simulink model "ControleLateralApplication_atual"  (R2023b)
settings: Solver=ode23tb  StartTime=0.0  StopTime=TME.Simulation  FixedStep=.001  RelTol=2e-1  EnableMultiTasking=on
StartFcn:
  | %tic
StopFcn:
  | %toc
model workspace (MAT data in the model file):
  A_mu = 10
  B_reff = 8.386
  Cz = 7766.25
  DCT_Param : object (value not decoded)
  DLCXref = [0 6 7 14 33.5 34 42 50 60]
  DLCYref = [0 0 -4.5 -4 -3.75 1.5 0.5 0 0]
  D_reff = 0.25826
  Downshift_Speeds = [9.5625 12.9375 16.3125 19.6875 23.0625 26.4375 29.8125 33.1875 36.5625 39.9375 43.3125 46.6875 ... (28 elements, 4x7)]
  EngRevLim = 7000
  Pedal_Positions = [0.1 0.4 0.5 0.9]
  SUS : object (value not decoded)
  Upshift_Speeds = [12.9375 16.3125 19.6875 33 26.4375 29.8125 33.1875 52.5 39.9375 43.3125 46.6875 77.25 ... (28 elements, 4x7)]
  VEH : object (value not decoded)
  V_o = 16.7
  V_xlow = 1
  WH : object (value not decoded)
  a = 1.4
  alpha_max = 1.5
  alpha_min = -1.5
  b = 1.8
  c_zo = 209651
  epsilon = 0.1
  h = 0.134
  path : object (value not decoded)
  pio = 220000
  q_Fcx = 0
  q_Fz2 = 15.4
  q_Fzy = 0
  q_reo = 0.9974
  q_sx1 = -0.007764
  q_sx10 = 0.2824
  q_sx11 = 5.349
  q_sx12 = 0
  q_sx13 = 0
  q_sx14 = 0
  q_sx2 = 1.1915
  q_sx3 = 0.013948
  q_sx4 = 4.912
  q_sx5 = 1.02
  q_sx6 = 22.83
  q_sx7 = 0.7104
  q_sx8 = -0.023393
  q_sx9 = 0.6581
  q_sy1 = 0.00702
  q_sy2 = 0
  q_sy3 = 0.001515
  q_sy4 = 8.514e-05
  q_sy5 = 0
  q_sy6 = 0
  q_sy7 = 0.9008
  q_sy8 = -0.4089
  q_v1 = 0.0007742
  q_v2 = 0.04667
  r_Bx1 = 12.531
  r_Bx2 = 9.532
  r_Bx3 = 0
  r_By1 = 10.615
  r_By2 = 7.705
  r_By3 = 3.433e-06
  r_By4 = 0
  r_Cx1 = 1.019
  r_Cy1 = 1.0585
  r_Ex1 = -0.4487
  r_Ex2 = -0.4726
  r_Ey1 = 0.3132
  r_Ey2 = 7.63e-06
  r_Hx1 = 0.0002374
  r_Hy1 = 0.011646
  r_Hy2 = 7.63e-06
  r_Vy1 = 0.05654
  r_Vy2 = 7.63e-06
  r_Vy3 = 0
  r_Vy4 = 99.9
  r_Vy5 = 2
  r_Vy6 = 15.814
  r_o = 0.3135
  vehWidth = 2
  w = 1
symbols that are objects in the model workspace (value not decoded): VEH
undefined symbols (not defined in the file): C1, C2, C3, Disabled, EV, GND, MTR, Right, SENSOR, STEER, WHL
libraries: autolibutils x5, vehdynlibscenariocommon x5, autolibshared x5, sim3dlib x4, vehdynlibtirecommon x2, autolibmappedmotor x2, vehdynlibviscommon x2, vehdynlibsteering x1, slpidlib x1, vehdynlibdriver x1, vehdynlibsens x1, sharedtransform x1
(part 6 of 6)

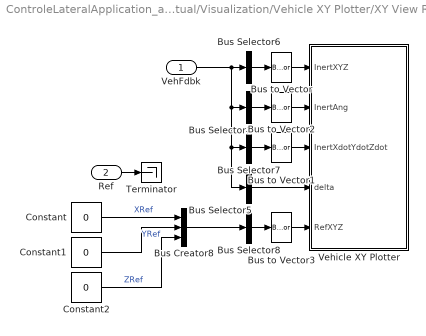
== system ControleLateralApplication_atual/Visualization/Vehicle XY Plotter/XY View Ref ==
  VehFdbk : Inport
  Ref : Inport  Port=2
  Bus Creator8 : BusCreator  Inputs=3
  Bus Selector1 : BusSelector  OutputSignals=Chassis.phi,Chassis.theta,Chassis.psi  OutputAsBus=on
  Bus Selector5 : BusSelector  OutputSignals=Driveline.WhlAng  OutputAsBus=on
  Bus Selector6 : BusSelector  OutputSignals=Chassis.GeomX,Chassis.GeomY,Chassis.GeomZ  OutputAsBus=on
  Bus Selector7 : BusSelector  OutputSignals=Chassis.GeomXdot,Chassis.GeomYdot,Chassis.GeomZdot  OutputAsBus=on
  Bus Selector8 : BusSelector  OutputSignals=XRef,YRef,ZRef  OutputAsBus=on
  Bus to Vector{,1..3} (4 alike) : BusToVector
  Constant : Constant  Value=0
  Constant1 : Constant  Value=0
  Constant2 : Constant  Value=0
  Terminator : Terminator
  Vehicle XY Plotter : Subsystem  mask(Vehicle XY Plotter){a=EV.FrontAxlePositionfromCG, b=EV.RearAxlePositionfromCG, w=EV.TrackWidth(1), figBorder=10, bufferSize=1024, extRef=on, pltDT=.1}
      mask prompts: a "Distance to front axle from CG, a [m]:"; b "Distance to rear axle from CG, b [m]:"; w "Track width, w [m]:"; figBorder "Distance to figure borders, figBorder [m]:"; bufferSize "Path buffer sampe size, bufferSize []:"; extRef "Plot path reference, extRef"; pltDT "Plot update rate, pltDT [s]:"
      mask help:
      | This block will display a MATLAB figure which indicates the vehicle path, current position and heading velocity.
      | An optional path reference is also provided.
      mask init: same as ControleLateralApplication_atual/Visualization/Vehicle XY Plotter/XY View/Vehicle XY Plotter
      mask TypeOptions a: Vehicle XY Plotter/a
      mask TypeOptions b: Vehicle XY Plotter/b
      mask TypeOptions w: Vehicle XY Plotter/w
      mask TypeOptions figBorder: Vehicle XY Plotter/figBorder
      mask TypeOptions bufferSize: Vehicle XY Plotter/bufferSize
  wires:
  Bus Selector8/1 -> Bus to Vector3/1
  Bus to Vector1/1 -> Vehicle XY Plotter/3(InertXdotYdotZdot)
  VehFdbk/1 -> Bus Selector5/1, Bus Selector7/1, Bus Selector1/1, Bus Selector6/1
  Bus Selector7/1 -> Bus to Vector1/1
  Bus Selector6/1 -> Bus to Vector/1
  Bus Selector1/1 -> Bus to Vector2/1
  Bus Selector5/1 -> Vehicle XY Plotter/4(delta)
  Bus to Vector/1 -> Vehicle XY Plotter/1(InertXYZ)
  Bus to Vector2/1 -> Vehicle XY Plotter/2(InertAng)
  Bus to Vector3/1 -> Vehicle XY Plotter/5(RefXYZ)
  Constant/1 -> Bus Creator8/1  "XRef"
  Constant1/1 -> Bus Creator8/2  "YRef"
  Constant2/1 -> Bus Creator8/3  "ZRef"
  Bus Creator8/1 -> Bus Selector8/1
  Ref/1 -> Terminator/1

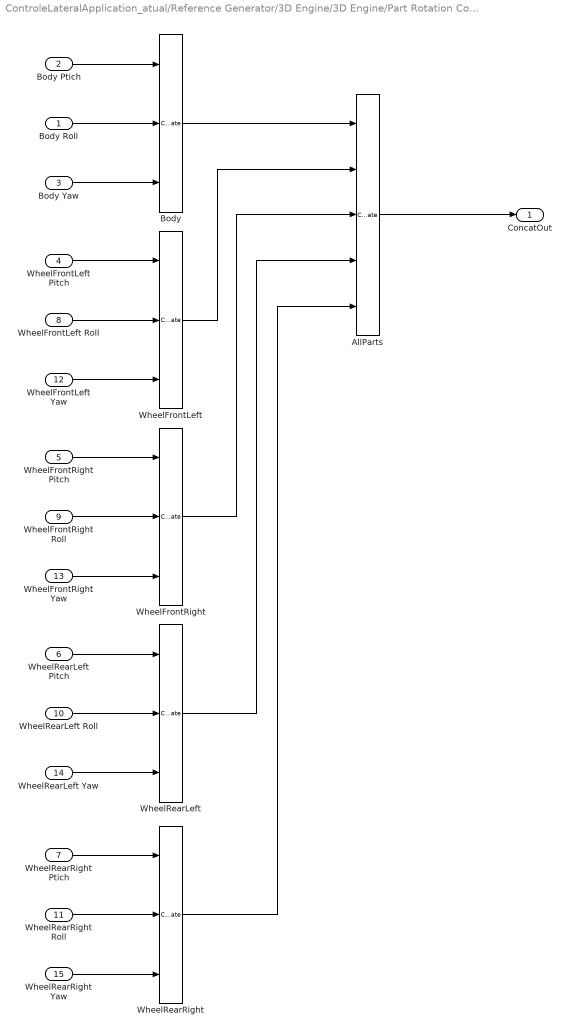
== system ControleLateralApplication_atual/Reference Generator/3D Engine/3D Engine/Part Rotation Concatenation ==
  Body Roll : Inport
  Body Ptich : Inport  Port=2
  Body Yaw : Inport  Port=3
  WheelFrontLeft Pitch : Inport  Port=4
  WheelFrontRight Pitch : Inport  Port=5
  WheelRearLeft Pitch : Inport  Port=6
  WheelRearRight Ptich : Inport  Port=7
  WheelFrontLeft Roll : Inport  Port=8
  WheelFrontRight Roll : Inport  Port=9
  WheelRearLeft Roll : Inport  Port=10
  WheelRearRight Roll : Inport  Port=11
  WheelFrontLeft Yaw : Inport  Port=12
  WheelFrontRight Yaw : Inport  Port=13
  WheelRearLeft Yaw : Inport  Port=14
  WheelRearRight Yaw : Inport  Port=15
  AllParts : Concatenate  NumInputs=5  Mode=Multidimensional array
  Body : Concatenate  NumInputs=3  Mode=Multidimensional array  ConcatenateDimension=2
  WheelFrontLeft : Concatenate  NumInputs=3  Mode=Multidimensional array  ConcatenateDimension=2
  WheelFrontRight : Concatenate  NumInputs=3  Mode=Multidimensional array  ConcatenateDimension=2
  WheelRearLeft : Concatenate  NumInputs=3  Mode=Multidimensional array  ConcatenateDimension=2
  WheelRearRight : Concatenate  NumInputs=3  Mode=Multidimensional array  ConcatenateDimension=2
  ConcatOut : Outport  VectorParamsAs1DForOutWhenUnconnected=off
  wires:
  Body Ptich/1 -> Body/1
  Body Yaw/1 -> Body/3
  WheelFrontLeft Pitch/1 -> WheelFrontLeft/1
  WheelFrontLeft Yaw/1 -> WheelFrontLeft/3
  WheelFrontLeft Roll/1 -> WheelFrontLeft/2
  Body Roll/1 -> Body/2
  WheelFrontLeft/1 -> AllParts/2
  WheelRearRight Ptich/1 -> WheelRearRight/1
  Body/1 -> AllParts/1
  WheelRearLeft/1 -> AllParts/4
  WheelFrontRight/1 -> AllParts/3
  WheelRearRight Yaw/1 -> WheelRearRight/3
  WheelFrontRight Roll/1 -> WheelFrontRight/2
  WheelFrontRight Pitch/1 -> WheelFrontRight/1
  WheelRearRight Roll/1 -> WheelRearRight/2
  WheelRearLeft Yaw/1 -> WheelRearLeft/3
  AllParts/1 -> ConcatOut/1
  WheelRearLeft Roll/1 -> WheelRearLeft/2
  WheelRearRight/1 -> AllParts/5
  WheelRearLeft Pitch/1 -> WheelRearLeft/1
  WheelFrontRight Yaw/1 -> WheelFrontRight/3

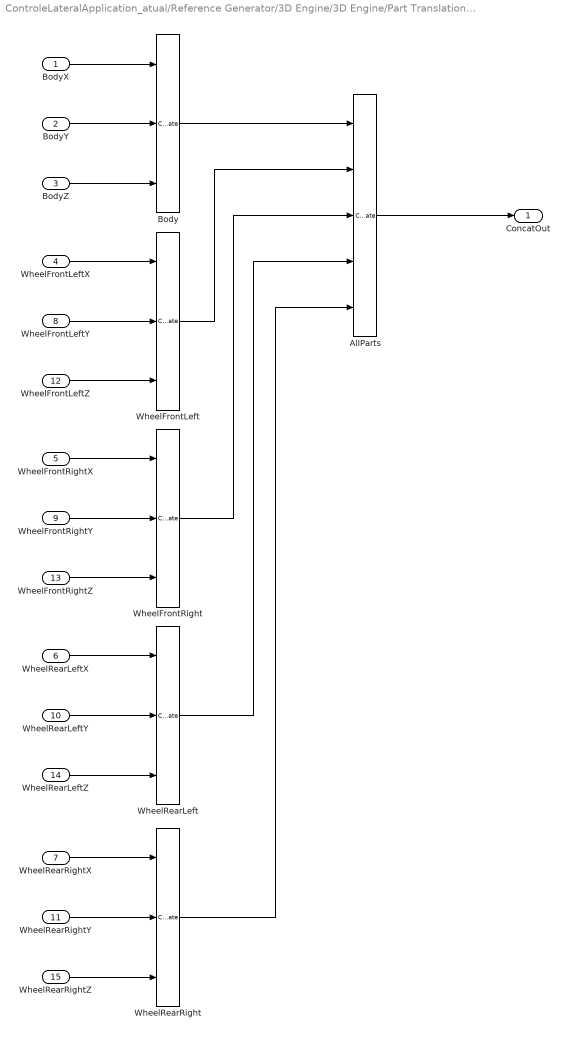
== system ControleLateralApplication_atual/Reference Generator/3D Engine/3D Engine/Part Translation Concatenation ==
  BodyX : Inport
  BodyY : Inport  Port=2
  BodyZ : Inport  Port=3
  WheelFrontLeftX : Inport  Port=4
  WheelFrontRightX : Inport  Port=5
  WheelRearLeftX : Inport  Port=6
  WheelRearRightX : Inport  Port=7
  WheelFrontLeftY : Inport  Port=8
  WheelFrontRightY : Inport  Port=9
  WheelRearLeftY : Inport  Port=10
  WheelRearRightY : Inport  Port=11
  WheelFrontLeftZ : Inport  Port=12
  WheelFrontRightZ : Inport  Port=13
  WheelRearLeftZ : Inport  Port=14
  WheelRearRightZ : Inport  Port=15
  AllParts : Concatenate  NumInputs=5  Mode=Multidimensional array
  Body : Concatenate  NumInputs=3  Mode=Multidimensional array  ConcatenateDimension=2
  WheelFrontLeft : Concatenate  NumInputs=3  Mode=Multidimensional array  ConcatenateDimension=2
  WheelFrontRight : Concatenate  NumInputs=3  Mode=Multidimensional array  ConcatenateDimension=2
  WheelRearLeft : Concatenate  NumInputs=3  Mode=Multidimensional array  ConcatenateDimension=2
  WheelRearRight : Concatenate  NumInputs=3  Mode=Multidimensional array  ConcatenateDimension=2
  ConcatOut : Outport  VectorParamsAs1DForOutWhenUnconnected=off
  wires:
  BodyX/1 -> Body/1
  BodyZ/1 -> Body/3
  WheelFrontLeftX/1 -> WheelFrontLeft/1
  WheelFrontLeftZ/1 -> WheelFrontLeft/3
  WheelFrontLeftY/1 -> WheelFrontLeft/2
  BodyY/1 -> Body/2
  WheelFrontLeft/1 -> AllParts/2
  WheelRearRightX/1 -> WheelRearRight/1
  Body/1 -> AllParts/1
  WheelRearLeft/1 -> AllParts/4
  WheelFrontRight/1 -> AllParts/3
  WheelRearRightZ/1 -> WheelRearRight/3
  WheelFrontRightY/1 -> WheelFrontRight/2
  WheelFrontRightX/1 -> WheelFrontRight/1
  WheelRearRightY/1 -> WheelRearRight/2
  WheelRearLeftZ/1 -> WheelRearLeft/3
  AllParts/1 -> ConcatOut/1
  WheelRearLeftY/1 -> WheelRearLeft/2
  WheelRearRight/1 -> AllParts/5
  WheelRearLeftX/1 -> WheelRearLeft/1
  WheelFrontRightZ/1 -> WheelFrontRight/3

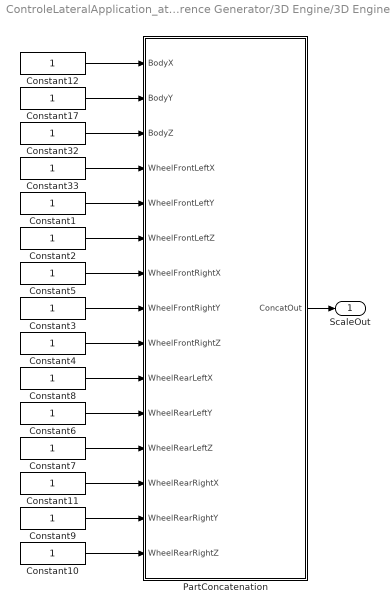
== system ControleLateralApplication_atual/Reference Generator/3D Engine/3D Engine/Scale ==
  Constant{1..12,17,32..33} (15 alike) : Constant  OutDataTypeStr=single
  PartConcatenation : Subsystem
  ScaleOut : Outport  VectorParamsAs1DForOutWhenUnconnected=off
  wires:
  Constant10/1 -> PartConcatenation/15(WheelRearRightZ)
  Constant9/1 -> PartConcatenation/14(WheelRearRightY)
  Constant11/1 -> PartConcatenation/13(WheelRearRightX)
  Constant7/1 -> PartConcatenation/12(WheelRearLeftZ)
  Constant6/1 -> PartConcatenation/11(WheelRearLeftY)
  Constant8/1 -> PartConcatenation/10(WheelRearLeftX)
  Constant4/1 -> PartConcatenation/9(WheelFrontRightZ)
  Constant3/1 -> PartConcatenation/8(WheelFrontRightY)
  Constant5/1 -> PartConcatenation/7(WheelFrontRightX)
  Constant2/1 -> PartConcatenation/6(WheelFrontLeftZ)
  Constant1/1 -> PartConcatenation/5(WheelFrontLeftY)
  Constant33/1 -> PartConcatenation/4(WheelFrontLeftX)
  Constant32/1 -> PartConcatenation/3(BodyZ)
  Constant17/1 -> PartConcatenation/2(BodyY)
  Constant12/1 -> PartConcatenation/1(BodyX)
  PartConcatenation/1(ConcatOut) -> ScaleOut/1

== system ControleLateralApplication_atual/Reference Generator/3D Engine/3D Engine/VehicleActorTransform 2 ==
  Constant : Constant  Value=[0 0 depth; 0 0 0; 0 0 0; 0 0 0; 0 0 0]
  Constant1 : Constant  Value=[0 0 0; 0 0 0; 0 0 0; 0 0 0; 0 0 0]
  Constant2 : Constant  Value=ones(5,3)
  Vehicle Actor Transform Set1 : sim3dlib/Simulation 3D Actor Transform Set  ActorTag=SimulinkVehicle2  NumberOfParts=5  CustNumOfParts=3  Translation=[0 0 depth; 0 0 0; 0 0 0; 0 0 0; 0 0 0]  Rotation=[0 0 0; 0 0 0; 0 0 0; 0 0 0; 0 0 0]  Scale=[1 1 1; 1 1 1; 1 1 1; 1 1 1; 1 1 1]  Ts=-1  aMode=aMode
  wires:
  Constant/1 -> Vehicle Actor Transform Set1/1
  Constant2/1 -> Vehicle Actor Transform Set1/3
  Constant1/1 -> Vehicle Actor Transform Set1/2

== system ControleLateralApplication_atual/Visualization/Vehicle XY Plotter/XY View/Vehicle XY Plotter ==
  InertXYZ : Inport
  InertAng : Inport  Port=2
  InertXdotYdotZdot : Inport  Port=3
  delta : Inport  Port=4
  Rate Transition{1..5} (5 alike) : RateTransition  Deterministic=off  OutPortSampleTime=pltDT
  RefXYZ Ground : Ground
  Vehicle XY Plotter : vehdynlibviscommon/Vehicle XY Plotter  w=w  a=a  b=b  figBorder=figBorder  bufferSize=bufferSize  extStats=off  extTireF=off
  wires:
  Rate Transition5/1 -> Vehicle XY Plotter/4
  Rate Transition4/1 -> Vehicle XY Plotter/3
  Rate Transition2/1 -> Vehicle XY Plotter/2
  Rate Transition1/1 -> Vehicle XY Plotter/1
  Rate Transition3/1 -> Vehicle XY Plotter/5
  delta/1 -> Rate Transition5/1  "delta"
  InertXYZ/1 -> Rate Transition1/1  "InertCGDisp"
  InertXdotYdotZdot/1 -> Rate Transition4/1  "InertCGVel"
  InertAng/1 -> Rate Transition2/1  "InertCGDisp"
  RefXYZ Ground/1 -> Rate Transition3/1

== system ControleLateralApplication_atual/Visualization/Vehicle XY Plotter/XY View Ref/Vehicle XY Plotter ==
  InertXYZ : Inport
  InertAng : Inport  Port=2
  InertXdotYdotZdot : Inport  Port=3
  delta : Inport  Port=4
  RefXYZ : Inport  Port=5
  Rate Transition{1..5} (5 alike) : RateTransition  Deterministic=off  OutPortSampleTime=pltDT
  Vehicle XY Plotter : vehdynlibviscommon/Vehicle XY Plotter  w=w  a=a  b=b  figBorder=figBorder  bufferSize=bufferSize  extStats=off  extTireF=off
  wires:
  InertAng/1 -> Rate Transition2/1  "InertCGDisp"
  InertXdotYdotZdot/1 -> Rate Transition4/1  "InertCGVel"
  InertXYZ/1 -> Rate Transition1/1  "InertCGDisp"
  delta/1 -> Rate Transition5/1  "delta"
  Rate Transition3/1 -> Vehicle XY Plotter/5
  Rate Transition1/1 -> Vehicle XY Plotter/1
  Rate Transition2/1 -> Vehicle XY Plotter/2
  Rate Transition4/1 -> Vehicle XY Plotter/3
  Rate Transition5/1 -> Vehicle XY Plotter/4
  RefXYZ/1 -> Rate Transition3/1

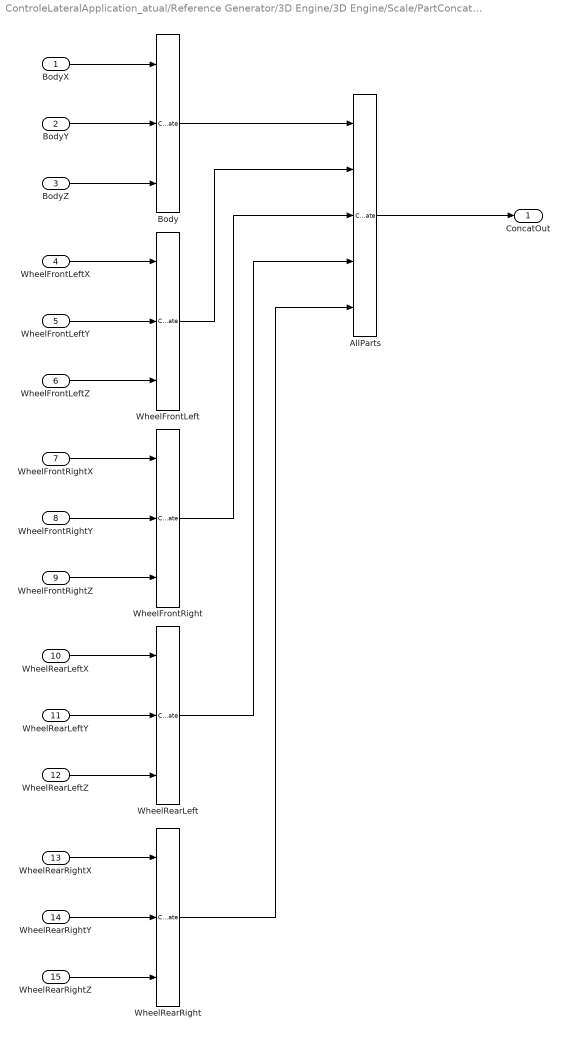
== system ControleLateralApplication_atual/Reference Generator/3D Engine/3D Engine/Scale/PartConcatenation ==
  BodyX : Inport
  BodyY : Inport  Port=2
  BodyZ : Inport  Port=3
  WheelFrontLeftX : Inport  Port=4
  WheelFrontLeftY : Inport  Port=5
  WheelFrontLeftZ : Inport  Port=6
  WheelFrontRightX : Inport  Port=7
  WheelFrontRightY : Inport  Port=8
  WheelFrontRightZ : Inport  Port=9
  WheelRearLeftX : Inport  Port=10
  WheelRearLeftY : Inport  Port=11
  WheelRearLeftZ : Inport  Port=12
  WheelRearRightX : Inport  Port=13
  WheelRearRightY : Inport  Port=14
  WheelRearRightZ : Inport  Port=15
  AllParts : Concatenate  NumInputs=5  Mode=Multidimensional array
  Body : Concatenate  NumInputs=3  Mode=Multidimensional array  ConcatenateDimension=2
  WheelFrontLeft : Concatenate  NumInputs=3  Mode=Multidimensional array  ConcatenateDimension=2
  WheelFrontRight : Concatenate  NumInputs=3  Mode=Multidimensional array  ConcatenateDimension=2
  WheelRearLeft : Concatenate  NumInputs=3  Mode=Multidimensional array  ConcatenateDimension=2
  WheelRearRight : Concatenate  NumInputs=3  Mode=Multidimensional array  ConcatenateDimension=2
  ConcatOut : Outport  VectorParamsAs1DForOutWhenUnconnected=off
  wires:
  BodyX/1 -> Body/1
  BodyZ/1 -> Body/3
  WheelFrontLeftX/1 -> WheelFrontLeft/1
  WheelFrontLeftZ/1 -> WheelFrontLeft/3
  WheelFrontLeftY/1 -> WheelFrontLeft/2
  BodyY/1 -> Body/2
  WheelFrontLeft/1 -> AllParts/2
  WheelRearRightX/1 -> WheelRearRight/1
  Body/1 -> AllParts/1
  WheelRearLeft/1 -> AllParts/4
  WheelFrontRight/1 -> AllParts/3
  WheelRearRightZ/1 -> WheelRearRight/3
  WheelFrontRightY/1 -> WheelFrontRight/2
  WheelFrontRightX/1 -> WheelFrontRight/1
  WheelRearRightY/1 -> WheelRearRight/2
  WheelRearLeftZ/1 -> WheelRearLeft/3
  AllParts/1 -> ConcatOut/1
  WheelRearLeftY/1 -> WheelRearLeft/2
  WheelRearRight/1 -> AllParts/5
  WheelRearLeftX/1 -> WheelRearLeft/1
  WheelFrontRightZ/1 -> WheelFrontRight/3

== matlab function ControleLateralApplication_atual/Cálculo do Skidpad ==
  settings: updateMethod=DISCRETE
  data: Angle input; Dist input; Diam output; Temp output; Vel input
% Calcula o diametro do circulo e o tempo gasto em uma volta, a partir da
% distância percorrida quando o veículo está entre 180 graus e 540 graus.
% É preciso fazer um interpolação devido a frequencia dos dados.
function [Diam,Temp] = fcn(Angle,Dist,Vel)

persistent Temp2
persistent Diam2
persistent DistA
persistent DistA1
persistent AngleA1
persistent DistB1
persistent AngleB1
persistent endA1
persistent endB1
persistent Start

if isempty(DistA1)
    Start = 2*pi; %define o valor que começa a marcação
    Diam2=0;
    Temp2=0;
    DistA=0;
    DistA1=0;
    AngleA1=0;
    DistB1=0;
    AngleB1=0;
    endA1=false;
    endB1=false;
end
if (Angle < 0)
    Angle=-Angle;
end
%Guarda o último valor da distância percorrida e do ângulo antes do carro
%realizar 180 graus
if(Angle < Start)
    AngleA1=Angle;
    DistA1=Dist;
end
%Guarda a distancia percorrida até o veículo realizar 180 graus a partir de
%uma interpolação com os valores imediatamente antes e depois do veículo
%realizar 180 graus.
if(Angle >= Start && ~endA1)
    XA=[AngleA1, Angle];
    VA=[DistA1,Dist];
    DistA=interp1(XA,VA,Start);
    endA1=true;
end
%Guarda o último valor da distância percorrida e do ângulo antes do carro
%realizar 540 graus
if(Angle < (2*pi + Start))
    AngleB1=Angle;
    DistB1=Dist;
end
%Calcula o diametro a partir da diferença entre a distancia percorrida até
%o veículo realizar 180 graus e a distancia percorrida até o veículo
%realizar 540 graus.
if(Angle >= (2*pi+Start) && ~endB1)
    XB=[AngleB1, Angle];
    VB=[DistB1,Dist];
    Diam2=(interp1(XB,VB,2*pi+Start) - DistA)/pi;
    Temp2=(interp1(XB,VB,2*pi+Start) - DistA)/Vel;
    endB1=true;
end
%iguala a variável de saida com a variável persistente.
Diam=Diam2;
Temp=Temp2;
end

== matlab function ControleLateralApplication_atual/For 3D Visualization ==
  data: angles output size=3; angleIn input size=3; GeomXYZ output size=3; GemoXYZIn input size=3; GroundZ input size=4; trackW parameter; wheelB parameter
function [angles,GeomXYZ]= three26(angleIn, GemoXYZIn, GroundZ,trackW, wheelB)%#codegen
coder.allowpcode('plain')
% Copyright 2018 The MathWorks, Inc.
[angles,GeomXYZ]= vdynthree2six(angleIn, GemoXYZIn, GroundZ,trackW, wheelB);

== matlab function ControleLateralApplication_atual/Kinematic Steering V2 ==
  data: Steer input; AngL output; AngR output; DadosVolante input; DadosE input; DadosD input
function [AngL,AngR]= fcn(Steer,DadosVolante,DadosE,DadosD)

AngL = (interp1(DadosVolante,DadosE,Steer));
AngR = (interp1(DadosVolante,DadosD,Steer));

== matlab function ControleLateralApplication_atual/le_acelerador ==
  data: APPS1 input; acelerador output
function acelerador = fcn(APPS1)

if (APPS1 >= 260 && APPS1 < 467)
    acelerador = (1.162 * APPS1 - 342.9);
    
else if (APPS1 >= 467 && APPS1 < 1065)
        acelerador = (0.3344 * APPS1 + 43.8);
        
    else if (APPS1 >= 1065 && APPS1 < 2253)
            acelerador = (0.1684 * APPS1 + 220.7);
            
        else if (APPS1 >= 2253 && APPS1 < 3211)
                acelerador = (0.2087 * APPS1 + 129.9);
                
            else if (APPS1 >= 3211 && APPS1 < 3720)
                    acelerador = (0.6598 * APPS1 - 1319);
                    
                else if (APPS1 >= 3720)
                        acelerador = 0;
                    else
                        acelerador = 0;
                    end
                end
            end
        end
    end
end
end

== matlab function ControleLateralApplication_atual/SKIDPAD Function ==
  data: x output; y output; theta output; psi input
% Cria um percurso do tipo Skidpad.

function [x,y,theta] = fcn(psi)

% CUIDADO
% x e y estão invertidos.

radius = 7.625;

%%
t = -psi + pi/9;
t1 = -t;

%% X, Y
xs = radius * cos(t) - radius;
ys = radius * sin(t);

%% Saídas
x = ys;
y = xs;
theta = t1;

end

== matlab function ControleLateralApplication_atual/SLALOM Function ==
  data: x output; y output; theta output; X_ input; Y_ input; psi input
% Cria um percurso do tipo Slalom.

function [x,y,theta] = fcn(X_, Y_, psi)

% CUIDADO
% X_ e Y_ estão invertidos.
% x e y estão invertidos.

xs = Y_ + pi/2; %pi/2
ys = sin(xs/5); %xs/4

if (ys >= 0)
    t1 = psi + 0.1;
else
    t1 = psi - 0.1;
end

%% Saídas
x = ys;
y = xs;
theta = t1;

end

== matlab function ControleLateralApplication_atual/Cálculo do Slalom ==
  settings: updateMethod=DISCRETE
  data: X_ input; Y_ input; Temp output; Vel input; R output
% Calcula o tempo gasto em um percurso slalom de 100m, a partir da
% distância percorrida entre Y_ = 180 e Y_ = 280.
% É importante observar que x e y estão invertidos.
function [Temp,R]  = fcn(X_,Y_,Vel)

persistent Temp2
persistent R1;
persistent R2;
persistent DistA
persistent DistB
persistent endA1
persistent endB1
persistent Start

if isempty(DistA)
    Start = 180; %define o valor que começa a marcação
    Temp2=0;
    R1 = 0;
    R2 = 0;
    DistA=0;
    DistB=0;
    endA1=false;
    endB1=false;
end
%Guarda o último valor da distância percorrida antes do carro atingir
%180m no eixo x.
if(Y_ < Start)
    DistA=Y_;
end
%Guarda o último valor da distância percorrida antes do carro atingir
%280m no eixo x.
if(Y_ >= Start && Y_ < (Start + 100))
    DistB=Y_;
    R1 = X_;
    %Guarda o valor maximo de Y atingido pelo carro.
    if (R1 > R2)
        R2 = R1;
    end
end
%Calcula o tempo a partir da diferença entre a distancia percorrida até
%o veículo atingir 180m e a distancia percorrida até o veículo atingir
%280m.
if(Y_ >= (Start + 100) && ~endB1)
    Temp2=(DistB - DistA)/Vel;
    endB1=true;
end
%iguala a variável de saida com a variável persistente.
Temp=Temp2;
R=R2;

end
